simulink model "linearizeDrone_motorcmdTostate"  (R2015a)
settings: Solver=ode45  StartTime=0.0  StopTime=10.0  RelTol=1e-3
InitFcn:
  | % load parameters of the default quadrotor
  | disp('Quadrotor parameters loaded by InitFcn')
  | paramsFilters %load mdl_quadcopter as well!
undefined symbols (not defined in the file or in its folder): quad, quadEDT
settings Model: Creator=ra  LastModifiedBy=ra

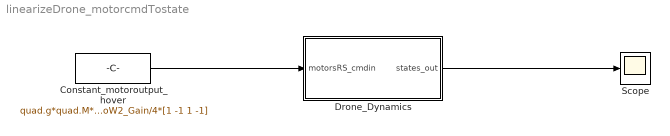
== system linearizeDrone_motorcmdTostate ==
  Constant_motoroutput_hover : Constant  Value=quad.g*quad.M*1/(quad.Ct*quad.rho*quad.A*quad.r^2)*1/quadEDT.motorsRSToW2_Gain/4*[1 -1 1 -1]
  Drone_Dynamics : Subsystem
  Scope : Scope
  wires:
  Constant_motoroutput_hover/1 -> Drone_Dynamics/1(motorsRS_cmdin)
  Drone_Dynamics/1(states_out) -> Scope/1

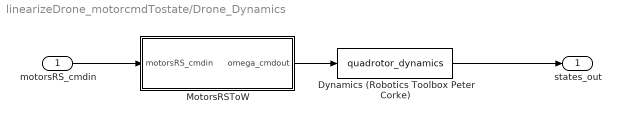
== system linearizeDrone_motorcmdTostate/Drone_Dynamics ==
  motorsRS_cmdin : Inport
  Dynamics (Robotics Toolbox Peter Corke) : S-Function  FunctionName=quadrotor_dynamics  Parameters=quad
  MotorsRSToW : Subsystem
  states_out : Outport
  wires:
  Dynamics (Robotics Toolbox Peter Corke)/1 -> states_out/1
  MotorsRSToW/1(omega_cmdout) -> Dynamics (Robotics Toolbox Peter Corke)/1
  motorsRS_cmdin/1 -> MotorsRSToW/1(motorsRS_cmdin)

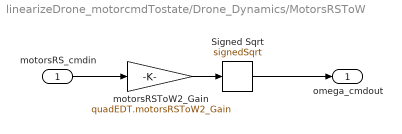
== system linearizeDrone_motorcmdTostate/Drone_Dynamics/MotorsRSToW ==
  motorsRS_cmdin : Inport
  Signed Sqrt : Sqrt  Operator=signedSqrt  SaturateOnIntegerOverflow=on
  motorsRSToW2_Gain : Gain  Gain=quadEDT.motorsRSToW2_Gain
  omega_cmdout : Outport
  wires:
  motorsRSToW2_Gain/1 -> Signed Sqrt/1
  motorsRS_cmdin/1 -> motorsRSToW2_Gain/1
  Signed Sqrt/1 -> omega_cmdout/1
